simulink model "EHB_speedgoat_R2020a_V1"  (R2020a)
settings: Solver=FixedStepDiscrete  StartTime=0.0  StopTime=inf  FixedStep=0.001  RelTol=1e-3  EnableMultiTasking=on
model workspace (MAT data in the model file):
  A : Simulink.Signal (value not decoded)
  B : Simulink.Signal (value not decoded)
  C : Simulink.Signal (value not decoded)
  D : Simulink.Signal (value not decoded)
  E : Simulink.Signal (value not decoded)
  calin = [-9.96 -7.98 -5.98 -3.99 -1.994 0 1.995 3.992 5.99 7.98 9.97]
  calout = [-10 -8 -6 -4 -2 0 2 4 6 8 10]
symbols that are objects in the model workspace (value not decoded): C, D
undefined symbols (not defined in the file): Com1, none, ts_IO612
libraries: simulink x1436, xpcethercatlib x1223, yisutbxlib_utilities x256, xpcutilitieslib x156, hdlsllib x145, canmsglib x46, speedgoatlib_IO602_4 x11, speedgoatlib_IO611 x7, slrttcplib x4, CanManageLib x3, slrtlib x3, xpcseriallib x2
(part 2 of 30)

== system EHB_speedgoat_R2020a_V1/TIF_04/CB2020_3 ==
  12V_DAC_CH1 : Constant  Commented=on  Value=0  OutDataTypeStr=Inherit: Inherit via back propagation
  ADC : Subsystem  mask(simucat_adc){deviceID=0, boxNum=Box 7 (Analog Board), channel1=off, channel2=off, channel3=off, channel4=off, channel5=on, channel6=off, channel7=off, channel8=off, channel9=off, channel10=off, channel11=off, channel12=off, channel13=off, channel14=off, channel15=off, channel16=off}
      mask prompts: deviceID "Device Index:"; boxNum "Select a box:"; channel1 "1"; channel2 "2"; channel3 "3"; channel4 "4"; channel5 "5"; channel6 "6"; channel7 "7"; channel8 "8"; channel9 "9"; channel10 "10"; channel11 "11"; channel12 "12"; channel13 "13"; channel14 "14"; channel15 "15"; channel16 "16"
      mask help:
      | SimuCat系列模拟板卡驱动模块。
      | 功能：模拟量转换数字量。通道数：16
      mask TypeOptions deviceID: 0 | 1 | 2 | 3 | 4 | 5 | 6 | 7 | 8 | 9 | 10 | 11 | 12 | 13 | 14 | 15
      mask TypeOptions boxNum: Box 5 (Analog Board) | Box 6 (Analog Board) | Box 7 (Analog Board)
      mask DialogControl refreshButton Prompt: Refresh
      mask DialogControl refreshButton Callback: ystbx.mask.callbacks.refreshBoxList
      mask DialogControl selectChannel Prompt: Select channels:
      mask DialogControl Dummy Prompt: (Add text here)
      mask DialogControl channelSelectAll Prompt: Select All
      mask DialogControl channelSelectAll Callback: ystbx.mask.callbacks.selectAllChannels();
      mask DialogControl channelClearAll Prompt: Clear All
      mask DialogControl channelClearAll Callback: ystbx.mask.callbacks.clearAllChannels();
      mask DialogControl applyButton Prompt: Apply Modification
      mask DialogControl applyButton Callback: ystbx.mask.callbacks.maskApply();
      mask Display: disp('CB2020(Analog Board)\nanalog-to-digital converter\nNetwork Device 0\nBox 7 (Analog Board)');port_label('output',1,'ADC_CH5[V]');
  ADC_CH{6..16} (11 alike) : Gain  Commented=on  OutDataTypeStr=Inherit: Inherit via back propagation
  ADC_CH5 : Gain  OutDataTypeStr=Inherit: Inherit via back propagation
  AI1 : Subsystem  Commented=on
  AI2 : Subsystem  Commented=on
  AI3 : Subsystem  Commented=on
  AI4 : Subsystem  Commented=on
  DAC1 : Subsystem  mask(simucat_dac){deviceID=0, boxNum=Box 7 (Analog Board), channel1=on, channel2=off, channel3=off, channel4=off, channel5=off, channel6=off, channel7=off, channel8=off, channel9=off, channel10=off, channel11=off, channel12=off, channel13=off, channel14=off, channel15=off, channel16=off, channel17=off, channel18=off, channel19=off, channel20=off, calEnable=off, currentMode=off}
      mask prompts: deviceID "Device Index:"; boxNum "Select a box:"; channel1 "1"; channel2 "2"; channel3 "3"; channel4 "4"; channel5 "5"; channel6 "6"; channel7 "7"; channel8 "8"; channel9 "9"; channel10 "10"; channel11 "11"; channel12 "12"; channel13 "13"; channel14 "14"; channel15 "15"; channel16 "16"; channel17 "17"; channel18 "18"; channel19 "19"; channel20 "20"; calEnable "Enable DAC Calibrate"; currentMode "Apply Last 4 Channels(17~20) with Current Mode"
      mask help:
      | SimuCat系列模拟板卡驱动模块。
      | 功能：数字量转换模拟量。通道数：20
      settings: OpenFcn=open_system(gcb, 'mask');
      mask TypeOptions deviceID: 0 | 1 | 2 | 3 | 4 | 5 | 6 | 7 | 8 | 9 | 10 | 11 | 12 | 13 | 14 | 15
      mask TypeOptions boxNum: Box 5 (Analog Board) | Box 6 (Analog Board) | Box 7 (Analog Board)
      mask DialogControl refreshButton Prompt: Refresh
      mask DialogControl refreshButton Callback: ystbx.mask.callbacks.refreshBoxList
      mask DialogControl selectChannel Prompt: Select channels:
      mask DialogControl Dummy Prompt: (Add text here)
      mask DialogControl channelSelectAll Prompt: Select All
      mask DialogControl channelSelectAll Callback: ystbx.mask.callbacks.selectAllChannels();
      mask DialogControl channelClearAll Prompt: Clear All
      mask DialogControl channelClearAll Callback: ystbx.mask.callbacks.clearAllChannels();
      mask DialogControl applyButton Prompt: Apply Modification
      mask DialogControl applyButton Callback: ystbx.mask.callbacks.maskApply();
      mask Display: disp('CB2020(Analog Board)\ndigital-to-analog converter\nNetwork Device 0\nBox 7 (Analog Board)');port_label('input',1,'DAC_CH1[V]');
  Divide : Product  Inputs=*/
  Gain : Gain
  Gain{1..15} (15 alike) : Gain  Commented=on
  K : Constant  Value=6
  Sw : Subsystem
  Sw1 : Subsystem  Commented=on
  Sw10 : Subsystem  Commented=on
  Sw11 : Subsystem  Commented=on
  Sw2 : Subsystem  Commented=on
  Sw3 : Subsystem  Commented=on
  Sw4 : Subsystem  Commented=on
  Sw5 : Subsystem  Commented=on
  Sw6 : Subsystem  Commented=on
  Sw7 : Subsystem  Commented=on
  Sw8 : Subsystem  Commented=on
  Sw9 : Subsystem  Commented=on
  Terminator : Terminator
  Terminator{1..15} (15 alike) : Terminator  Commented=on
  mean1 : Subsystem
  mean10 : Subsystem  Commented=on
  mean11 : Subsystem  Commented=on
  mean12 : Subsystem  Commented=on
  mean13 : Subsystem  Commented=on
  mean14 : Subsystem  Commented=on
  mean15 : Subsystem  Commented=on
  mean16 : Subsystem  Commented=on
  mean2 : Subsystem  Commented=on
  mean3 : Subsystem  Commented=on
  mean4 : Subsystem  Commented=on
  mean5 : Subsystem  Commented=on
  mean6 : Subsystem  Commented=on
  mean7 : Subsystem  Commented=on
  mean8 : Subsystem  Commented=on
  mean9 : Subsystem  Commented=on
  tag scope: Power_5V=global
  wires:
  ADC_CH10/1 -> Gain5/1  "ADC_CH10"
  ADC_CH8/1 -> Gain3/1  "ADC_CH8"
  ADC_CH14/1 -> Gain9/1  "ADC_CH14"
  ADC_CH5/1 -> [Power_5V], Gain/1  "ADC_CH5"
  ADC_CH12/1 -> Gain7/1  "ADC_CH12"
  ADC_CH16/1 -> Gain11/1  "ADC_CH16"
  ADC_CH15/1 -> Gain10/1  "ADC_CH15"
  ADC_CH7/1 -> Gain2/1  "ADC_CH7"
  ADC_CH11/1 -> Gain6/1  "ADC_CH11"
  ADC_CH13/1 -> Gain8/1  "ADC_CH13"
  ADC_CH6/1 -> Gain1/1  "ADC_CH6"
  ADC_CH9/1 -> Gain4/1  "ADC_CH9"
  AI4/1(Cur) -> Gain15/1  "ADC_CH24"
  AI3/1(Cur) -> Gain14/1  "ADC_CH23"
  AI2/1(Cur) -> Gain13/1  "ADC_CH22"
  AI1/1(Cur) -> Gain12/1  "ADC_CH21"
  mean16/1(Vol) -> AI4/1(Vol)
  mean15/1(Vol) -> AI3/1(Vol)
  mean14/1(Vol) -> AI2/1(Vol)
  mean13/1(Vol) -> AI1/1(Vol)
  mean1/1(Vol) -> Sw/3(Vol), Sw/1(In2), Sw/2(In3)
  Sw/1(Out1) -> ADC_CH5/1
  mean2/1(Vol) -> Sw1/3(Vol), Sw1/1(In2), Sw1/2(In3)
  mean3/1(Vol) -> Sw2/3(Vol), Sw2/2(In3), Sw2/1(In2)
  mean4/1(Vol) -> Sw3/3(Vol), Sw3/2(In3), Sw3/1(In2)
  mean5/1(Vol) -> Sw4/3(Vol), Sw4/2(In3), Sw4/1(In2)
  mean6/1(Vol) -> Sw5/3(Vol), Sw5/2(In3), Sw5/1(In2)
  mean7/1(Vol) -> Sw6/3(Vol), Sw6/2(In3), Sw6/1(In2)
  mean8/1(Vol) -> Sw7/3(Vol), Sw7/2(In3), Sw7/1(In2)
  mean9/1(Vol) -> Sw9/3(Vol), Sw9/2(In3), Sw9/1(In2)
  mean10/1(Vol) -> Sw8/3(In3), Sw8/2(In2), Sw8/1(Vol)
  mean11/1(Vol) -> Sw10/3(Vol), Sw10/2(In3), Sw10/1(In2)
  mean12/1(Vol) -> Sw11/3(Vol), Sw11/2(In3), Sw11/1(In2)
  Sw11/1(Out1) -> ADC_CH16/1
  Sw10/1(Out1) -> ADC_CH15/1
  Sw8/1(Out1) -> ADC_CH14/1
  Sw9/1(Out1) -> ADC_CH13/1
  Sw7/1(Out1) -> ADC_CH12/1
  Sw6/1(Out1) -> ADC_CH11/1
  Sw5/1(Out1) -> ADC_CH10/1
  Sw4/1(Out1) -> ADC_CH9/1
  Sw3/1(Out1) -> ADC_CH8/1
  Sw2/1(Out1) -> ADC_CH7/1
  Sw1/1(Out1) -> ADC_CH6/1
  ADC/1(ADC_CH5[V]) -> mean1/1(In1)
  Gain/1 -> Terminator/1
  Gain1/1 -> Terminator1/1
  Gain2/1 -> Terminator2/1
  Gain3/1 -> Terminator3/1
  Gain4/1 -> Terminator4/1
  Gain5/1 -> Terminator5/1
  Gain11/1 -> Terminator11/1
  Gain10/1 -> Terminator10/1
  Gain9/1 -> Terminator9/1
  Gain8/1 -> Terminator8/1
  Gain7/1 -> Terminator7/1
  Gain6/1 -> Terminator6/1
  Gain15/1 -> Terminator15/1
  Gain14/1 -> Terminator14/1
  Gain13/1 -> Terminator13/1
  Gain12/1 -> Terminator12/1
  K/1 -> Divide/2
  [PowerOn_Off] -> Divide/1  "12V_DAC_CH1"
  Divide/1 -> DAC1/1(DAC_CH1[V])  "12V_DAC_CH1"

== system EHB_speedgoat_R2020a_V1/YS5002/YS5002_M_PowerCtrl ==
  note: 1、模拟量控制比例要看具体电源输出范围计算，
      |      例如：电源0~80V对应DAC的0~10V，设定12V时实际下发给DAC的是1/8*1000mV。
      | 2、Rly通过哪两个继电器去控制KL30,15要确认下机柜具体的实际接线，一般是Rly1,2。
      | 3、OnOff一般接SwitchA，通过下降沿去触发。
  YS5002_M : Inport
  Enable : EnablePort
  Bus Selector : BusSelector  OutputSignals=PS1,PS2,PS3,PS4
  CAN Pack : canmsglib/CAN Pack  MsgList=(none)  MsgName=PowerSet  MsgIDType=Standard (11-bit identifier)  MsgIdentifier=1852  MsgLength=8  Remote=off  ApplyMinMax=off  BusOutput=on  SignalInfo={ 'ADC1_Calibration_en', '52', '1', 'BE', 'unsigned', 'Standard', '0', '1', '0', '0', '1'; 'ADC2_Calibration_en', '53', '1', 'BE', 'unsigned', 'Standard', '0', '1', '0', '0', '1'; 'ADCorDAC_Calibration_Data', '56', '12', 'BE', 'unsigned', 'Standard', '0', '1', '0', '500', '1500'; 'Calibration_en', '14', '1', 'BE', 'unsigned', 'Standard', '0', '1', '0', '0', '1'; 'DAC1_Set', '24', '16', 'BE', 'unsigned', 'Standard', '0', '1', '0', '0', '10000'; 'DAC2_Set', '40', '16', 'BE', 'unsigned', 'Standard', '0', '1', '0', '0', '10000'; 'DCA1_Calibration_en', '54', '1', 'BE', 'unsigned', 'Standard', '0', '1', '0', '0', '1'; 'DCA2_Calibration_en', '55', '1', 'BE', 'unsigned', 'Standard', '0', '1', '0', '0', '1'; 'Rly1_Ctrl', '11', '1', 'BE', 'unsigned', 'Standard', '0', '1', '0', '0', '1'; 'Rly2_Ctrl', '10', '1', 'BE', 'unsigned', 'Standard', '0', '1', '0', '0', '1'; 'Rly3_Ctrl', '9', '1', 'BE', 'unsigned', 'Standard', '0', '1', '0', '0', '1'; 'Rly4_Ctrl', '8', '1', 'BE', 'unsigned', 'Standard', '0', '1', '0', '0', '1'; 'Slot', '0', '8', 'BE', 'unsigned', 'Standard', '0', '1', '0', '0', '15'; 'SwitchA', '12', '1', 'BE', 'unsigned', 'Standard', '0', '1', '0', '0', '1'; 'SwitchB', '13', '1', 'BE', 'unsigned', 'Standard', '0', '1', '0', '0', '1'; 'Trig_en', '15', '1', 'BE', 'unsigned', 'Standard', '0', '1', '0', '0', '1' }
      settings: SourceProductBaseCode=ME,XP,VN  DataFormat=manually specified signals
  CANDataPack_ToUDP : Subsystem
  Cur : Constant  Value=0  OutDataTypeStr=Inherit: Inherit via back propagation
  Gain1 : Gain  Gain=1000/8
  Gain2 : Gain  Gain=1000/8
  InternalUse : Constant  Value=0  OutDataTypeStr=Inherit: Inherit via back propagation
  InternalUse1 : Constant  Value=0  OutDataTypeStr=Inherit: Inherit via back propagation
  Logical Operator : Logic  Operator=NOT  AllPortsSameDT=off  OutDataTypeStr=boolean
  Solt : Constant  Value=0
  Sw : Constant  Value=0  OutDataTypeStr=Inherit: Inherit via back propagation
  SwitchB : Constant  Value=0  OutDataTypeStr=Inherit: Inherit via back propagation
  Trig_en : Constant  Value=0  OutDataTypeStr=Inherit: Inherit via back propagation
  Vol : Constant  Value=0  OutDataTypeStr=Inherit: Inherit via back propagation
  Output : Outport
  wires:
  Vol/1 -> Gain2/1  "VoltSet"
  Cur/1 -> Gain1/1  "CurrLimSet"
  InternalUse/1 -> CAN Pack/4, CAN Pack/3, CAN Pack/2, CAN Pack/1
  YS5002_M/1 -> Bus Selector/1
  Bus Selector/1 -> [PS1]  "<PS1>"
  Bus Selector/2 -> [PS2]  "<PS2>"
  Bus Selector/3 -> [PS3]  "<PS3>"
  Solt/1 -> CAN Pack/13
  [PS1] -> CAN Pack/9
  [PS2] -> CAN Pack/10
  Trig_en/1 -> CAN Pack/16  "Trig_en"
  Gain2/1 -> CAN Pack/5  "DAC1_Set"
  Gain1/1 -> CAN Pack/6  "DAC2_Set"
  InternalUse1/1 -> CAN Pack/8, CAN Pack/7
  Bus Selector/4 -> [PS4]  "<PS4>"
  SwitchB/1 -> CAN Pack/14
  Logical Operator/1 -> CAN Pack/15
  Sw/1 -> Logical Operator/1  "Sw"
  [PS3] -> CAN Pack/11
  [PS4] -> CAN Pack/12
  CAN Pack/1 -> CANDataPack_ToUDP/1(In1)
  CANDataPack_ToUDP/1(Out1) -> Output/1

== system EHB_speedgoat_R2020a_V1/保留/IO602 ==
  CAN Pack : canmsglib/CAN Pack  MsgList=(none)  MsgName=CAN Msg  MsgIDType=Standard (11-bit identifier)  MsgIdentifier=100  MsgLength=8  Remote=off  ApplyMinMax=off  BusOutput=off  SignalInfo={'Signal1','0','64','LE','double','Standard','0','1','0','-Inf','Inf'}
      settings: SourceProductBaseCode=ME,VN  DataFormat=manually specified signals
  CAN Pack1 : canmsglib/CAN Pack  MsgList=(none)  MsgName=CAN Msg  MsgIDType=Standard (11-bit identifier)  MsgIdentifier=101  MsgLength=8  Remote=off  ApplyMinMax=off  BusOutput=off  SignalInfo={'Signal1','0','64','LE','double','Standard','0','1','0','-Inf','Inf'}
      settings: SourceProductBaseCode=ME,VN  DataFormat=manually specified signals
  CAN Pack2 : canmsglib/CAN Pack  MsgList=(none)  MsgName=CAN Msg  MsgIDType=Standard (11-bit identifier)  MsgIdentifier=102  MsgLength=8  Remote=off  ApplyMinMax=off  BusOutput=off  SignalInfo={'Signal1','0','64','LE','double','Standard','0','1','0','-Inf','Inf'}
      settings: SourceProductBaseCode=ME,VN  DataFormat=manually specified signals
  CAN Pack3 : canmsglib/CAN Pack  MsgList=(none)  MsgName=CAN Msg  MsgIDType=Standard (11-bit identifier)  MsgIdentifier=100  MsgLength=8  Remote=off  ApplyMinMax=off  BusOutput=off  SignalInfo={'Signal1','0','64','LE','double','Standard','0','1','0','-Inf','Inf'}
      settings: SourceProductBaseCode=ME,VN  DataFormat=manually specified signals
  CAN Pack4 : canmsglib/CAN Pack  MsgList=(none)  MsgName=CAN Msg  MsgIDType=Standard (11-bit identifier)  MsgIdentifier=101  MsgLength=8  Remote=off  ApplyMinMax=off  BusOutput=off  SignalInfo={'Signal1','0','64','LE','double','Standard','0','1','0','-Inf','Inf'}
      settings: SourceProductBaseCode=ME,VN  DataFormat=manually specified signals
  CAN Pack5 : canmsglib/CAN Pack  MsgList=(none)  MsgName=CAN Msg  MsgIDType=Standard (11-bit identifier)  MsgIdentifier=102  MsgLength=8  Remote=off  ApplyMinMax=off  BusOutput=off  SignalInfo={'Signal1','0','64','LE','double','Standard','0','1','0','-Inf','Inf'}
      settings: SourceProductBaseCode=ME,VN  DataFormat=manually specified signals
  CAN Read Loop - Port 1 : Subsystem  TreatAsAtomicUnit=on
  CAN Read Loop - Port 3 : Subsystem  TreatAsAtomicUnit=on
  CAN Write : speedgoatlib_IO602_4/Legacy/CAN Write  id=1  ts=-1  channel=1  messageType=CAN  BusInput=off  enableStatusPort=off  canType=CAN (HS)  initValues=[602 1 -1 0 1 1 0 0]
      settings: SourceProductName=Simulink Real-Time: Speedgoat I/O Blockset
  CAN Write1 : speedgoatlib_IO602_4/Legacy/CAN Write  id=1  ts=-1  channel=1  messageType=CAN  BusInput=off  enableStatusPort=off  canType=CAN (HS)  initValues=[602 1 -1 0 1 1 0 0]
      settings: SourceProductName=Simulink Real-Time: Speedgoat I/O Blockset
  CAN Write2 : speedgoatlib_IO602_4/Legacy/CAN Write  id=1  ts=-1  channel=1  messageType=CAN  BusInput=off  enableStatusPort=off  canType=CAN (HS)  initValues=[602 1 -1 0 1 1 0 0]
      settings: SourceProductName=Simulink Real-Time: Speedgoat I/O Blockset
  CAN Write3 : speedgoatlib_IO602_4/Legacy/CAN Write  id=1  ts=-1  channel=3  messageType=CAN  BusInput=off  enableStatusPort=off  canType=CAN (HS)  initValues=[602 1 -1 2 1 1 0 0]
      settings: SourceProductName=Simulink Real-Time: Speedgoat I/O Blockset
  CAN Write4 : speedgoatlib_IO602_4/Legacy/CAN Write  id=1  ts=-1  channel=3  messageType=CAN  BusInput=off  enableStatusPort=off  canType=CAN (HS)  initValues=[602 1 -1 2 1 1 0 0]
      settings: SourceProductName=Simulink Real-Time: Speedgoat I/O Blockset
  CAN Write5 : speedgoatlib_IO602_4/Legacy/CAN Write  id=1  ts=-1  channel=3  messageType=CAN  BusInput=off  enableStatusPort=off  canType=CAN (HS)  initValues=[602 1 -1 2 1 1 0 0]
      settings: SourceProductName=Simulink Real-Time: Speedgoat I/O Blockset
  Mux : Mux  Inputs=3
  Mux2 : Mux  Inputs=3
  RX Sample Time : Constant  SampleTime=ts_IO612
  RX Sample Time1 : Constant  SampleTime=ts_IO612
  "Scope " : slrtlib/Displays and Logging/Scope   scopeno=1  scopetype=Target  autostart=on  viewmode=Graphical redraw  formatstr='%15.6f'  grid=on  ylimits=[0,0]  nosamples=250  noprepostsamples=0  interleave=1  triggermode=FreeRun  triggersignal=1  trigsignalfromport=off  triggerlevel=0.0  triggerslope=Rising  triggerscope=1  triggersample=0  filename=data.dat  mode=Lazy  writesize=512  autorestart=off  dynamicfilemode=off  maxwritefilesize=512*1024^2
  Scope 1 : slrtlib/Displays and Logging/Scope   scopeno=2  scopetype=Target  autostart=on  viewmode=Graphical redraw  formatstr='%15.6f'  grid=on  ylimits=[0,0]  nosamples=250  noprepostsamples=0  interleave=1  triggermode=FreeRun  triggersignal=1  trigsignalfromport=off  triggerlevel=0.0  triggerslope=Rising  triggerscope=1  triggersample=0  filename=data.dat  mode=Lazy  writesize=512  autorestart=off  dynamicfilemode=off  maxwritefilesize=512*1024^2
  Sine Wave : Sin  Amplitude=10  Frequency=2*pi*10  SampleTime=ts_IO612
  Sine Wave1 : Sin  Amplitude=20  Frequency=2*pi*10  SampleTime=ts_IO612
  Sine Wave2 : Sin  Amplitude=30  Frequency=2*pi*10  SampleTime=ts_IO612
  Sine Wave3 : Sin  Amplitude=10  Frequency=2*pi*10  SampleTime=ts_IO612
  Sine Wave4 : Sin  Amplitude=20  Frequency=2*pi*10  SampleTime=ts_IO612
  Sine Wave5 : Sin  Amplitude=30  Frequency=2*pi*10  SampleTime=ts_IO612
  wires:
  Mux/1 -> "Scope "/1  "IO602Can1-2"
  CAN Read Loop - Port 3/1(ID100_Signal1) -> Mux/1
  CAN Read Loop - Port 3/3(ID102_Signal1) -> Mux/3
  CAN Read Loop - Port 3/2(ID101_Signal1) -> Mux/2
  RX Sample Time/1 -> CAN Read Loop - Port 3/1(SampleTime)
  Sine Wave1/1 -> CAN Pack1/1
  Sine Wave/1 -> CAN Pack/1
  Sine Wave2/1 -> CAN Pack2/1
  CAN Pack/1 -> CAN Write/1
  CAN Pack1/1 -> CAN Write1/1
  CAN Pack2/1 -> CAN Write2/1
  CAN Pack5/1 -> CAN Write5/1
  CAN Pack4/1 -> CAN Write4/1
  CAN Pack3/1 -> CAN Write3/1
  Sine Wave5/1 -> CAN Pack5/1
  Sine Wave3/1 -> CAN Pack3/1
  Sine Wave4/1 -> CAN Pack4/1
  RX Sample Time1/1 -> CAN Read Loop - Port 1/1(SampleTime)
  CAN Read Loop - Port 1/2(ID101_Signal1) -> Mux2/2
  CAN Read Loop - Port 1/3(ID102_Signal1) -> Mux2/3
  CAN Read Loop - Port 1/1(ID100_Signal1) -> Mux2/1
  Mux2/1 -> Scope 1/1  "IO602Can3-4"

== system EHB_speedgoat_R2020a_V1/保留/IO611 ==
  note: PORT 1 - TX
  note: PORT 1 - TX
  note: PORT 2 - RX
  note: PORT 2 - RX
  "Byte Packing " : xpcutilitieslib/Byte Packing   MaskPackedDataType=uint8  MaskUnpackedDataTypes={'uint8','uint8'}  MaskAlignment=1
  CAN Pack : canmsglib/CAN Pack  MsgList=(none)  MsgName=CAN Msg  MsgIDType=Standard (11-bit identifier)  MsgIdentifier=100  MsgLength=8  Remote=off  ApplyMinMax=off  BusOutput=off  SignalInfo={'Signal1','0','64','LE','double','Standard','0','1','0','-Inf','Inf'}
      settings: SourceProductBaseCode=ME,VN  DataFormat=manually specified signals
  CAN Pack1 : canmsglib/CAN Pack  MsgList=(none)  MsgName=CAN Msg  MsgIDType=Standard (11-bit identifier)  MsgIdentifier=101  MsgLength=8  Remote=off  ApplyMinMax=off  BusOutput=off  SignalInfo={'Signal1','0','64','LE','double','Standard','0','1','0','-Inf','Inf'}
      settings: SourceProductBaseCode=ME,VN  DataFormat=manually specified signals
  CAN Pack2 : canmsglib/CAN Pack  MsgList=(none)  MsgName=CAN Msg  MsgIDType=Standard (11-bit identifier)  MsgIdentifier=102  MsgLength=8  Remote=off  ApplyMinMax=off  BusOutput=off  SignalInfo={'Signal1','0','64','LE','double','Standard','0','1','0','-Inf','Inf'}
      settings: SourceProductBaseCode=ME,VN  DataFormat=manually specified signals
  CAN Read Loop - Port 3 : Subsystem  TreatAsAtomicUnit=on
  CAN Write : speedgoatlib_IO611/Legacy/CAN/CAN Write  id=1  sampleTime=-1  portSelection=1  messageType=CAN  BusInput=off  enaStatusPort=off  protl=IO611  ptIdx=0  isFDMod=1
      settings: SourceProductName=Simulink Real-Time: Speedgoat I/O Blockset
  CAN Write1 : speedgoatlib_IO611/Legacy/CAN/CAN Write  id=1  sampleTime=-1  portSelection=1  messageType=CAN  BusInput=off  enaStatusPort=off  protl=IO611  ptIdx=0  isFDMod=1
      settings: SourceProductName=Simulink Real-Time: Speedgoat I/O Blockset
  CAN Write2 : speedgoatlib_IO611/Legacy/CAN/CAN Write  id=1  sampleTime=-1  portSelection=1  messageType=CAN  BusInput=off  enaStatusPort=off  protl=IO611  ptIdx=0  isFDMod=1
      settings: SourceProductName=Simulink Real-Time: Speedgoat I/O Blockset
  Constant1 : Constant  Value=80  OutDataTypeStr=uint8
  Data Type Conversion : DataTypeConversion
  Gain : Gain
  "LIN Master Write v2 " : speedgoatlib_IO611/Legacy/LIN/LIN Master Write v2   id=1  sampleTime=-1  portSelection=3  messageType=RAW  linVersion=LIN 2.X  protIdent=0  dlc=2  dummy1=dummy for default msg data used for slave write block  protl=IO611  ptIdx=2  isSlv=0  isEnhcdChksum=1  qtyMsgBlkLIN=1
      settings: SourceProductName=Simulink Real-Time: Speedgoat I/O Blockset
  "LIN Slave Read v2 " : speedgoatlib_IO611/Legacy/LIN/LIN Slave Read v2   id=1  sampleTime=-1  portSelection=4  enaUpdateState=off  enaMsgType=off  enaDataOverrun=off  enaTimeStampe=off  messageType=RAW  linVersion=LIN 2.X  protIdent=0  dlc=2  protl=IO611  ptIdx=3  isSlv=1  isEnhcdChksum=1  qtyMsgBlkLIN=1
      settings: SourceProductName=Simulink Real-Time: Speedgoat I/O Blockset
  Mux : Mux  Inputs=3
  Pulse Generator : DiscretePulseGenerator  PulseType=Time based  Amplitude=20  Period=10  PulseWidth=50
  RX Sample Time : Constant  SampleTime=ts_IO612
  "Scope " : slrtlib/Displays and Logging/Scope   scopeno=3  scopetype=Target  autostart=on  viewmode=Graphical redraw  formatstr='%15.6f'  grid=on  ylimits=[0,0]  nosamples=250  noprepostsamples=0  interleave=1  triggermode=FreeRun  triggersignal=1  trigsignalfromport=off  triggerlevel=0.0  triggerslope=Rising  triggerscope=1  triggersample=0  filename=data.dat  mode=Lazy  writesize=512  autorestart=off  dynamicfilemode=off  maxwritefilesize=512*1024^2
  Sine Wave : Sin  Amplitude=10  Frequency=2*pi*10  SampleTime=ts_IO612
  Sine Wave1 : Sin  Amplitude=20  Frequency=2*pi*10  SampleTime=ts_IO612
  Sine Wave2 : Sin  Amplitude=30  Frequency=2*pi*10  SampleTime=ts_IO612
  Terminator : Terminator
  wires:
  Constant1/1 -> "Byte Packing "/1  "LIN_Data1"
  Pulse Generator/1 -> Data Type Conversion/1
  "Byte Packing "/1 -> "LIN Master Write v2 "/1
  "LIN Slave Read v2 "/1 -> Gain/1  "IO611_LIN_Rx"
  CAN Pack1/1 -> CAN Write1/1
  Sine Wave2/1 -> CAN Pack2/1
  Sine Wave/1 -> CAN Pack/1
  CAN Read Loop - Port 3/3(ID102_Signal1) -> Mux/3
  Sine Wave1/1 -> CAN Pack1/1
  RX Sample Time/1 -> CAN Read Loop - Port 3/1(SampleTime)
  CAN Pack2/1 -> CAN Write2/1
  CAN Read Loop - Port 3/2(ID101_Signal1) -> Mux/2
  CAN Pack/1 -> CAN Write/1
  CAN Read Loop - Port 3/1(ID100_Signal1) -> Mux/1
  Mux/1 -> "Scope "/1  "IO611"
  Data Type Conversion/1 -> "Byte Packing "/2  "LIN_Data2"
  Gain/1 -> Terminator/1

== system EHB_speedgoat_R2020a_V1/保留/RS232 ==
  Baseboard Serial F2 : xpcseriallib/Mainboard/Baseboard Serial F  group=FIFO Setup  port=1  irqnum=4  saddr1=0x3f8  saddr2=0x3e8  config=Com1/none  baud1=115200  parity1=None  ndata1=8  nstop1=1  fifomode1=16 deep  rlevel1=half full  automode1=on  xmtfifosize1=1024  xmtdatatype1=count+16 bit uint  rcvfifosize1=1024  baud2=115200  parity2=None  ndata2=8  nstop2=1  fifomode2=16 deep  rlevel2=half full  automode2=off  xmtfifosize2=1024  xmtdatatype2=8 bit uint null terminated  rcvfifosize2=1024
      settings: SourceProductBaseCode=XP
  "Byte Packing " : xpcutilitieslib/Byte Packing   MaskPackedDataType=uint8  MaskUnpackedDataTypes={'double'}  MaskAlignment=1
  Constant1 : Constant  Value=10
  Data Type Conversion : DataTypeConversion  OutDataTypeStr=uint16
  Data Type Conversion1 : DataTypeConversion  OutDataTypeStr=double
  "FIFO read " : xpcseriallib/FIFO read   maxsize=16  minsize=8  usedelimiter=off  delimiter=13  outputtype=count+16 bit uint  enable=off  enableout=off  sampletime=-1
      settings: SourceProductBaseCode=XP
  Gain : Gain
  Gain1 : Gain
  Ground3 : Ground
  Mux : Mux  Inputs=2
  Selector : Selector  InputPortWidth=17  IndexOptions=Index vector (dialog)  Indices=[2:9]  OutputSizes=1
  Terminator : Terminator
  Terminator1 : Terminator
  Terminator4 : Terminator
  Width : Width  DataType=uint16
  wires:
  "FIFO read "/1 -> Gain1/1, Selector/1  "FIOFO_Received_Data"
  Baseboard Serial F2/2 -> Terminator4/1
  Constant1/1 -> "Byte Packing "/1
  Ground3/1 -> Baseboard Serial F2/2
  Mux/1 -> Baseboard Serial F2/1  "RS232_Send"
  Width/1 -> Mux/1
  Data Type Conversion/1 -> Mux/2
  "Byte Packing "/1 -> Width/1, Data Type Conversion/1  "pack"
  Baseboard Serial F2/1 -> "FIFO read "/1
  Selector/1 -> Data Type Conversion1/1
  Data Type Conversion1/1 -> Gain/1  "RS232ReceiveData"
  Gain/1 -> Terminator/1
  Gain1/1 -> Terminator1/1

== system EHB_speedgoat_R2020a_V1/保留/TIF_01 ==
  YS4020_M_2 : Subsystem

== system EHB_speedgoat_R2020a_V1/保留/TIF_02 ==
  CB3012_01 : Subsystem

== system EHB_speedgoat_R2020a_V1/保留/TIF_03 ==
  CB1032_3 : Subsystem
  CB1032_4 : Subsystem

== system EHB_speedgoat_R2020a_V1/保留/TIF_06 ==
  CB1032_1 : Subsystem
  CB1032_2 : Subsystem
  YS4020_M_1 : Subsystem

== system EHB_speedgoat_R2020a_V1/保留/YS4008 ==
  YS4008_M_1 : Subsystem
  YS4008_M_2 : Subsystem
  YS4008_M_3 : Subsystem
  YS4008_M_4 : Subsystem
  YS4008_M_5 : Subsystem
  YS4008_M_6 : Subsystem

== system EHB_speedgoat_R2020a_V1/保留/YS7501_M ==
  Bitwise OR : simulink/Logic and Bit Operations/Bitwise Operator  logicop=OR  UseBitMask=off  BitMask=bin2dec('11011001')  BitMaskRealWorld=Stored Integer
  Constant{,1..15} (16 alike) : Constant  Value=0
  Detect Change : simulink/Logic and Bit Operations/Detect Change  vinit=0  OutDataTypeStr=boolean
  HVRealy_Set : Subsystem
  Mux : Mux  Inputs=16
  tag scope: YS7501_M=global
  wires:
  Constant1/1 -> HVRealy_Set/2(RLY2), Mux/2
  Constant3/1 -> HVRealy_Set/4(RLY4), Mux/4
  Constant2/1 -> HVRealy_Set/3(RLY3), Mux/3
  Constant/1 -> HVRealy_Set/1(RLY1), Mux/1
  Mux/1 -> Detect Change/1
  Constant4/1 -> HVRealy_Set/5(RLY5), Mux/5
  Constant5/1 -> HVRealy_Set/6(RLY6), Mux/6
  Constant7/1 -> HVRealy_Set/8(RLY8), Mux/8
  Constant8/1 -> HVRealy_Set/9(RLY9), Mux/9
  Constant9/1 -> HVRealy_Set/10(RLY10), Mux/10
  Constant10/1 -> HVRealy_Set/11(RLY11), Mux/11
  Constant11/1 -> HVRealy_Set/12(RLY12), Mux/12
  Constant12/1 -> HVRealy_Set/13(RLY13), Mux/13
  Constant13/1 -> Mux/14, HVRealy_Set/14(RLY14)
  Constant14/1 -> Mux/15, HVRealy_Set/15(RLY15)
  Constant15/1 -> Mux/16, HVRealy_Set/16(RLY16)
  Constant6/1 -> HVRealy_Set/7(RLY7), Mux/7
  Detect Change/1 -> Bitwise OR/1  "HVRealy_Ctrl_Trigger"
  Bitwise OR/1 -> HVRealy_Set/Trigger
  HVRealy_Set/1(Output) -> [YS7501_M]

== system EHB_speedgoat_R2020a_V1/CAN_Rec/CAN Receive/CAN_Msg_0x125 ==
  CAN Msg : Inport
  Enable : EnablePort
  Bus Creator : BusCreator  Inputs=6
  Can Unpack : canmsglib/CAN Unpack  CANdbFile=D:\Matlab\EHB_Prj\data\DBC\wushuadianji_20230612.dbc  MsgList=EHB_BrakingResponse  MsgName=EHB_BrakingResponse  MsgIDType=Standard (11-bit identifier)  MsgIdentifier=293  MsgLength=8  SignalInfo={'ActualPressure','8','8','BE','unsigned','Standard','0','0.1','0','-Inf','Inf';'BrakeCondition','1','2','BE','unsigned','Standard','0','1','0','-Inf','Inf';'Checksum','56','8','BE','unsigned','Standard','0','1','0','-Inf','Inf';'EHBFaultLevel','3','4','BE','unsigned','Standard','0','1','0','-Inf','Inf';'EHBStatus','0','1','BE','unsigned','Standard','0','1','0','-Inf','Inf';'RollingCounter','52','4','BE','unsigned','Standard','0','1','0','-Inf','Inf'}  IDPort=off  TimestampPort=off  ErrorPort=off  RemotePort=off  LengthPort=off  StatusPort=off  ApplyMinMax=off
      settings: SourceProductBaseCode=ME,VN  DataFormat=CANdb specified signals
  EHB_0125h_AliveCounter : DataTypeConversion
  EHB_0125h_CheckSUM : DataTypeConversion
  EHB_ActualPressure : DataTypeConversion
  EHB_BrakeCondition : DataTypeConversion
  EHB_EHBFaultLevel : DataTypeConversion
  EHB_Status : DataTypeConversion
  CAN_Msg_0x125 : Outport
  wires:
  Bus Creator/1 -> CAN_Msg_0x125/1  "CAN_Msg_0x125"
  EHB_0125h_CheckSUM/1 -> Bus Creator/3  "EHB_0125h_CheckSUM"
  Can Unpack/3 -> EHB_0125h_CheckSUM/1
  EHB_BrakeCondition/1 -> Bus Creator/2  "EHB_BrakeCondition"
  Can Unpack/2 -> EHB_BrakeCondition/1
  EHB_ActualPressure/1 -> Bus Creator/1  "EHB_ActualPressure"
  Can Unpack/1 -> EHB_ActualPressure/1
  CAN Msg/1 -> Can Unpack/1
  Can Unpack/4 -> EHB_EHBFaultLevel/1
  Can Unpack/5 -> EHB_Status/1
  Can Unpack/6 -> EHB_0125h_AliveCounter/1
  EHB_EHBFaultLevel/1 -> Bus Creator/4  "EHB_EHBFaultLevel"
  EHB_Status/1 -> Bus Creator/5  "EHB_Status"
  EHB_0125h_AliveCounter/1 -> Bus Creator/6  "EHB_0125h_AliveCounter"

== system EHB_speedgoat_R2020a_V1/CAN_Rec/CAN Receive/CAN_Msg_0x126 ==
  CAN Msg : Inport
  Enable : EnablePort
  Bus Creator : BusCreator  Inputs=22
  Can Unpack : canmsglib/CAN Unpack  CANdbFile=D:\Matlab\EHB_Prj\data\DBC\wushuadianji_20230612.dbc  MsgList=EHB_Diagnostics  MsgName=EHB_Diagnostics  MsgIDType=Standard (11-bit identifier)  MsgIdentifier=294  MsgLength=8  SignalInfo={'BrkReqWarn','0','1','BE','unsigned','Standard','0','1','0','-Inf','Inf';'CANBusOff','12','1','BE','unsigned','Standard','0','1','0','-Inf','Inf';'EHB_HardwareVersion','56','8','BE','unsigned','Standard','0','1','0','-Inf','Inf';'EHB_SoftwareVersion','48','8','BE','unsigned','Standard','0','1','0','-Inf','Inf';'ISnsrFlt','14','1','BE','unsigned','Standard','0','1','0','-Inf','Inf';'LoadMismatchFlt','11','1','BE','unsigned','Standard','0','1','0','-Inf','Inf';'MotPosnFlt','19','1','BE','unsigned','Standard','0','1','0','-Inf','Inf';'NTCFltLv1','3','1','BE','unsigned','Standard','0','1','0','-Inf','Inf';'NTCFltLv2','4','1','BE','unsigned','Standard','0','1','0','-Inf','Inf';'OverIFlt','13','1','BE','unsigned','Standard','0','1','0','-Inf','Inf';'OverTempWarn','6','1','BE','unsigned','Standard','0','1','0','-Inf','Inf';'PCtrlVibLv1','2','1','BE','unsigned','Standard','0','1','0','-Inf','Inf';'PCtrlVibLv2','10','1','BE','unsigned','Standard','0','1','0','-Inf','Inf';'PFolwFltLv1','1','1','BE','unsigned','Standard','0','1','0','-Inf','Inf';'PFolwFltLv2','9','1','BE','unsigned','Standard','0','1','0','-Inf','Inf';'PSnsrFlt','5','1','BE','unsigned','Standard','0','1','0','-Inf','Inf';'PwrDrvrFlt','18','1','BE','unsigned','Standard','0','1','0','-Inf','Inf';'PwrSwtFlt','17','1','BE','unsigned','Standard','0','1','0','-Inf','Inf';'USplyHighLv1','8','1','BE','unsigned','Standard','0','1','0','-Inf','Inf';'USplyHighLv2','16','1','BE','unsigned','Standard','0','1','0','-Inf','Inf';'USplyLowLv1','7','1','BE','unsigned','Standard','0','1','0','-Inf','Inf';'USplyLowLv2','15','1','BE','unsigned','Standard','0','1','0','-Inf','Inf'}  IDPort=off  TimestampPort=off  ErrorPort=off  RemotePort=off  LengthPort=off  StatusPort=off  ApplyMinMax=off
      settings: SourceProductBaseCode=ME,VN  DataFormat=CANdb specified signals
  EHB_BrkReqWarn : DataTypeConversion
  EHB_CANBusOff : DataTypeConversion
  EHB_HardwareVersion : DataTypeConversion
  EHB_ISnsrFlt : DataTypeConversion
  EHB_LoadMismatchFlt : DataTypeConversion
  EHB_MotPosnFlt : DataTypeConversion
  EHB_NTCFltLv1 : DataTypeConversion
  EHB_NTCFltLv2 : DataTypeConversion
  EHB_OverIFlt : DataTypeConversion
  EHB_OverTempWarn : DataTypeConversion
  EHB_PCtrlVibLv1 : DataTypeConversion
  EHB_PCtrlVibLv2 : DataTypeConversion
  EHB_PFolwFltLv1 : DataTypeConversion
  EHB_PFolwFltLv2 : DataTypeConversion
  EHB_PSnsrFlt : DataTypeConversion
  EHB_PwrDrvrFlt : DataTypeConversion
  EHB_PwrSwtFlt : DataTypeConversion
  EHB_SoftwareVersion : DataTypeConversion
  EHB_USplyHighLv1 : DataTypeConversion
  EHB_USplyHighLv2 : DataTypeConversion
  EHB_USplyLowLv1 : DataTypeConversion
  EHB_USplyLowLv2 : DataTypeConversion
  CAN_Msg_0x126 : Outport
  wires:
  EHB_LoadMismatchFlt/1 -> Bus Creator/6  "EHB_LoadMismatchFlt"
  EHB_ISnsrFlt/1 -> Bus Creator/5  "EHB_ISnsrFlt"
  EHB_SoftwareVersion/1 -> Bus Creator/4  "EHB_SoftwareVersion"
  Can Unpack/6 -> EHB_LoadMismatchFlt/1
  Can Unpack/5 -> EHB_ISnsrFlt/1
  Can Unpack/4 -> EHB_SoftwareVersion/1
  CAN Msg/1 -> Can Unpack/1
  Can Unpack/1 -> EHB_BrkReqWarn/1
  EHB_BrkReqWarn/1 -> Bus Creator/1  "EHB_BrkReqWarn"
  Can Unpack/2 -> EHB_CANBusOff/1
  EHB_CANBusOff/1 -> Bus Creator/2  "EHB_CANBusOff"
  Can Unpack/3 -> EHB_HardwareVersion/1
  EHB_HardwareVersion/1 -> Bus Creator/3  "EHB_HardwareVersion"
  Bus Creator/1 -> CAN_Msg_0x126/1  "CAN_Msg_0x126"
  Can Unpack/7 -> EHB_MotPosnFlt/1
  Can Unpack/8 -> EHB_NTCFltLv1/1
  Can Unpack/9 -> EHB_NTCFltLv2/1
  Can Unpack/10 -> EHB_OverIFlt/1
  Can Unpack/11 -> EHB_OverTempWarn/1
  Can Unpack/12 -> EHB_PCtrlVibLv1/1
  Can Unpack/13 -> EHB_PCtrlVibLv2/1
  Can Unpack/14 -> EHB_PFolwFltLv1/1
  Can Unpack/15 -> EHB_PFolwFltLv2/1
  Can Unpack/16 -> EHB_PSnsrFlt/1
  Can Unpack/17 -> EHB_PwrDrvrFlt/1
  Can Unpack/18 -> EHB_PwrSwtFlt/1
  Can Unpack/19 -> EHB_USplyHighLv1/1
  Can Unpack/20 -> EHB_USplyHighLv2/1
  Can Unpack/21 -> EHB_USplyLowLv1/1
  Can Unpack/22 -> EHB_USplyLowLv2/1
  EHB_MotPosnFlt/1 -> Bus Creator/7  "EHB_MotPosnFlt"
  EHB_NTCFltLv1/1 -> Bus Creator/8  "EHB_NTCFltLv1"
  EHB_NTCFltLv2/1 -> Bus Creator/9  "EHB_NTCFltLv2"
  EHB_OverIFlt/1 -> Bus Creator/10  "EHB_OverIFlt"
  EHB_OverTempWarn/1 -> Bus Creator/11  "EHB_OverTempWarn"
  EHB_PCtrlVibLv1/1 -> Bus Creator/12  "EHB_PCtrlVibLv1"
  EHB_PCtrlVibLv2/1 -> Bus Creator/13  "EHB_PCtrlVibLv2"
  EHB_PFolwFltLv1/1 -> Bus Creator/14  "EHB_PFolwFltLv1"
  EHB_PFolwFltLv2/1 -> Bus Creator/15  "EHB_PFolwFltLv2"
  EHB_PSnsrFlt/1 -> Bus Creator/16  "EHB_PSnsrFlt"
  EHB_PwrDrvrFlt/1 -> Bus Creator/17  "EHB_PwrDrvrFlt"
  EHB_PwrSwtFlt/1 -> Bus Creator/18  "EHB_PwrSwtFlt"
  EHB_USplyHighLv1/1 -> Bus Creator/19  "EHB_USplyHighLv1"
  EHB_USplyHighLv2/1 -> Bus Creator/20  "EHB_USplyHighLv2"
  EHB_USplyLowLv1/1 -> Bus Creator/21  "EHB_USplyLowLv1"
  EHB_USplyLowLv2/1 -> Bus Creator/22  "EHB_USplyLowLv2"

== system EHB_speedgoat_R2020a_V1/CAN_Rec/CAN Receive/CAN_Msg_0x127 ==
  CAN Msg : Inport
  Enable : EnablePort
  Bus Creator : BusCreator  Inputs=8
  Can Unpack : canmsglib/CAN Unpack  CANdbFile=D:\Matlab\EHB_Prj\data\DBC\wushuadianji_20230612.dbc  MsgList=EHB_WhlSpd_Info  MsgName=EHB_WhlSpd_Info  MsgIDType=Standard (11-bit identifier)  MsgIdentifier=295  MsgLength=8  SignalInfo={'WhlFLSpd','10','14','BE','unsigned','Standard','0','1','0','-Inf','Inf';'WhlFLSpdVld','8','2','BE','unsigned','Standard','0','1','0','-Inf','Inf';'WhlFRSpd','26','14','BE','unsigned','Standard','0','1','0','-Inf','Inf';'WhlFRSpdVld','24','2','BE','unsigned','Standard','0','1','0','-Inf','Inf';'WhlRLSpd','42','14','BE','unsigned','Standard','0','1','0','-Inf','Inf';'WhlRLSpdVld','40','2','BE','unsigned','Standard','0','1','0','-Inf','Inf';'WhlRRSpd','58','14','BE','unsigned','Standard','0','1','0','-Inf','Inf';'WhlRRSpdVld','56','2','BE','unsigned','Standard','0','1','0','-Inf','Inf'}  IDPort=off  TimestampPort=off  ErrorPort=off  RemotePort=off  LengthPort=off  StatusPort=off  ApplyMinMax=off
      settings: SourceProductBaseCode=ME,VN  DataFormat=CANdb specified signals
  EHB_WhlFLSpd : DataTypeConversion
  EHB_WhlFLSpdVld : DataTypeConversion
  EHB_WhlFRSpd : DataTypeConversion
  EHB_WhlFRSpdVld : DataTypeConversion
  EHB_WhlRLSpd : DataTypeConversion
  EHB_WhlRLSpdVld : DataTypeConversion
  EHB_WhlRRSpd : DataTypeConversion
  EHB_WhlRRSpdVld : DataTypeConversion
  CAN_Msg_0x127 : Outport
  wires:
  EHB_WhlRLSpdVld/1 -> Bus Creator/6  "EHB_WhlRLSpdVld"
  EHB_WhlRLSpd/1 -> Bus Creator/5  "EHB_WhlRLSpd"
  EHB_WhlFRSpdVld/1 -> Bus Creator/4  "EHB_WhlFRSpdVld"
  Can Unpack/6 -> EHB_WhlRLSpdVld/1
  Can Unpack/5 -> EHB_WhlRLSpd/1
  Can Unpack/4 -> EHB_WhlFRSpdVld/1
  CAN Msg/1 -> Can Unpack/1
  Can Unpack/1 -> EHB_WhlFLSpd/1
  EHB_WhlFLSpd/1 -> Bus Creator/1  "EHB_WhlFLSpd"
  Can Unpack/2 -> EHB_WhlFLSpdVld/1
  EHB_WhlFLSpdVld/1 -> Bus Creator/2  "EHB_WhlFLSpdVld"
  Can Unpack/3 -> EHB_WhlFRSpd/1
  EHB_WhlFRSpd/1 -> Bus Creator/3  "EHB_WhlFRSpd"
  Bus Creator/1 -> CAN_Msg_0x127/1  "CAN_Msg_0x127"
  Can Unpack/7 -> EHB_WhlRRSpd/1
  Can Unpack/8 -> EHB_WhlRRSpdVld/1
  EHB_WhlRRSpd/1 -> Bus Creator/7  "EHB_WhlRRSpd"
  EHB_WhlRRSpdVld/1 -> Bus Creator/8  "EHB_WhlRRSpdVld"

== system EHB_speedgoat_R2020a_V1/CAN_Rec/CAN Receive/Debug1_0x287 ==
  CAN Msg : Inport
  Enable : EnablePort
  Bus Creator : BusCreator  Inputs=4
  Can Unpack : canmsglib/CAN Unpack  CANdbFile=F:\湖大艾盛\wushuadianji_20230612.dbc  MsgList=Debug1  MsgName=Debug1  MsgIDType=Standard (11-bit identifier)  MsgIdentifier=647  MsgLength=8  SignalInfo={'iBeta','8','16','BE','signed','Standard','0','0.01','0','-Inf','Inf';'ia_ADC','40','16','BE','unsigned','Standard','0','1','0','-Inf','Inf';'ib_ADC','56','16','BE','unsigned','Standard','0','1','0','-Inf','Inf';'sin_theta','24','16','BE','signed','Standard','0','0.001','0','-Inf','Inf'}  IDPort=off  TimestampPort=off  ErrorPort=off  RemotePort=off  LengthPort=off  StatusPort=off  ApplyMinMax=off
      settings: SourceProductBaseCode=ME,VN  DataFormat=CANdb specified signals
  iBeta : DataTypeConversion
  ia_ADC : DataTypeConversion
  ib_ADC : DataTypeConversion
  sin_theta : DataTypeConversion
  Debug1 : Outport
  wires:
  CAN Msg/1 -> Can Unpack/1
  Can Unpack/1 -> iBeta/1
  iBeta/1 -> Bus Creator/1  "iBeta"
  Can Unpack/2 -> ia_ADC/1
  ia_ADC/1 -> Bus Creator/2  "ia_ADC"
  Can Unpack/3 -> ib_ADC/1
  ib_ADC/1 -> Bus Creator/3  "ib_ADC"
  Can Unpack/4 -> sin_theta/1
  sin_theta/1 -> Bus Creator/4  "sin_theta"
  Bus Creator/1 -> Debug1/1  "Debug1"

== system EHB_speedgoat_R2020a_V1/CAN_Rec/CAN Receive/Debug_0x286 ==
  CAN Msg : Inport
  Enable : EnablePort
  Bus Creator : BusCreator  Inputs=4
  Can Unpack : canmsglib/CAN Unpack  CANdbFile=F:\湖大艾盛\wushuadianji_20230612.dbc  MsgList=Debug  MsgName=Debug  MsgIDType=Standard (11-bit identifier)  MsgIdentifier=646  MsgLength=8  SignalInfo={'Ualpha','40','16','BE','signed','Standard','0','1','0','-Inf','Inf';'Ubeta','56','16','BE','signed','Standard','0','1','0','-Inf','Inf';'angle','8','16','BE','unsigned','Standard','0','1','0','-Inf','Inf';'cos_theta','24','16','BE','signed','Standard','0','0.001','0','-Inf','Inf'}  IDPort=off  TimestampPort=off  ErrorPort=off  RemotePort=off  LengthPort=off  StatusPort=off  ApplyMinMax=off
      settings: SourceProductBaseCode=ME,VN  DataFormat=CANdb specified signals
  Ualpha : DataTypeConversion
  Ubeta : DataTypeConversion
  angle : DataTypeConversion
  cos_theta : DataTypeConversion
  Debug : Outport
  wires:
  CAN Msg/1 -> Can Unpack/1
  Can Unpack/1 -> Ualpha/1
  Ualpha/1 -> Bus Creator/1  "Ualpha"
  Can Unpack/2 -> Ubeta/1
  Ubeta/1 -> Bus Creator/2  "Ubeta"
  Can Unpack/3 -> angle/1
  angle/1 -> Bus Creator/3  "angle"
  Can Unpack/4 -> cos_theta/1
  cos_theta/1 -> Bus Creator/4  "cos_theta"
  Bus Creator/1 -> Debug/1  "Debug"

== system EHB_speedgoat_R2020a_V1/CAN_Rec/CAN Receive/Message_1_0x281 ==
  CAN Msg : Inport
  Enable : EnablePort
  Angle1 : DataTypeConversion
  Bus Creator : BusCreator  Inputs=4
  Can Unpack : canmsglib/CAN Unpack  CANdbFile=F:\湖大艾盛\wushuadianji_20230612.dbc  MsgList=Message_1  MsgName=Message_1  MsgIDType=Standard (11-bit identifier)  MsgIdentifier=641  MsgLength=8  SignalInfo={'Angle1','56','16','BE','signed','Standard','0','1','0','-Inf','Inf';'U_Current','8','16','BE','signed','Standard','0','1','0','-Inf','Inf';'V_Current','24','16','BE','signed','Standard','0','1','0','-Inf','Inf';'W_Current','40','16','BE','signed','Standard','0','1','0','-Inf','Inf'}  IDPort=off  TimestampPort=off  ErrorPort=off  RemotePort=off  LengthPort=off  StatusPort=off  ApplyMinMax=off
      settings: SourceProductBaseCode=ME,VN  DataFormat=CANdb specified signals
  U_Current : DataTypeConversion
  V_Current : DataTypeConversion
  W_Current : DataTypeConversion
  Message_1 : Outport
  wires:
  CAN Msg/1 -> Can Unpack/1
  Can Unpack/1 -> Angle1/1
  Angle1/1 -> Bus Creator/1  "Angle1"
  Can Unpack/2 -> U_Current/1
  U_Current/1 -> Bus Creator/2  "U_Current"
  Can Unpack/3 -> V_Current/1
  V_Current/1 -> Bus Creator/3  "V_Current"
  Can Unpack/4 -> W_Current/1
  W_Current/1 -> Bus Creator/4  "W_Current"
  Bus Creator/1 -> Message_1/1  "Message_1"

== system EHB_speedgoat_R2020a_V1/CAN_Rec/CAN Receive/Message_2_0x282 ==
  CAN Msg : Inport
  Enable : EnablePort
  Angle2 : DataTypeConversion
  Bus Creator : BusCreator  Inputs=4
  Can Unpack : canmsglib/CAN Unpack  CANdbFile=F:\湖大艾盛\wushuadianji_20230612.dbc  MsgList=Message_2  MsgName=Message_2  MsgIDType=Standard (11-bit identifier)  MsgIdentifier=642  MsgLength=8  SignalInfo={'Angle2','8','16','BE','signed','Standard','0','1','0','-Inf','Inf';'U_DutyCycle','24','16','BE','signed','Standard','0','1','0','-Inf','Inf';'V_DutyCycle','40','16','BE','signed','Standard','0','1','0','-Inf','Inf';'W_DutyCycle','56','16','BE','signed','Standard','0','1','0','-Inf','Inf'}  IDPort=off  TimestampPort=off  ErrorPort=off  RemotePort=off  LengthPort=off  StatusPort=off  ApplyMinMax=off
      settings: SourceProductBaseCode=ME,VN  DataFormat=CANdb specified signals
  U_DutyCycle : DataTypeConversion
  V_DutyCycle : DataTypeConversion
  W_DutyCycle : DataTypeConversion
  Message_2 : Outport
  wires:
  CAN Msg/1 -> Can Unpack/1
  Can Unpack/1 -> Angle2/1
  Angle2/1 -> Bus Creator/1  "Angle2"
  Can Unpack/2 -> U_DutyCycle/1
  U_DutyCycle/1 -> Bus Creator/2  "U_DutyCycle"
  Can Unpack/3 -> V_DutyCycle/1
  V_DutyCycle/1 -> Bus Creator/3  "V_DutyCycle"
  Can Unpack/4 -> W_DutyCycle/1
  W_DutyCycle/1 -> Bus Creator/4  "W_DutyCycle"
  Bus Creator/1 -> Message_2/1  "Message_2"

== system EHB_speedgoat_R2020a_V1/CAN_Rec/CAN Receive/Message_3_0x283 ==
  CAN Msg : Inport
  Enable : EnablePort
  Bus Creator : BusCreator  Inputs=2
  Can Unpack : canmsglib/CAN Unpack  CANdbFile=F:\湖大艾盛\wushuadianji_20230612.dbc  MsgList=Message_3  MsgName=Message_3  MsgIDType=Standard (11-bit identifier)  MsgIdentifier=643  MsgLength=8  SignalInfo={'ia_act','24','32','BE','signed','Standard','0','1','0','-Inf','Inf';'ib_act','56','32','BE','signed','Standard','0','1','0','-Inf','Inf'}  IDPort=off  TimestampPort=off  ErrorPort=off  RemotePort=off  LengthPort=off  StatusPort=off  ApplyMinMax=off
      settings: SourceProductBaseCode=ME,VN  DataFormat=CANdb specified signals
  ia_act : DataTypeConversion
  ib_act : DataTypeConversion
  Message_3 : Outport
  wires:
  CAN Msg/1 -> Can Unpack/1
  Can Unpack/1 -> ia_act/1
  ia_act/1 -> Bus Creator/1  "ia_act"
  Can Unpack/2 -> ib_act/1
  ib_act/1 -> Bus Creator/2  "ib_act"
  Bus Creator/1 -> Message_3/1  "Message_3"

== system EHB_speedgoat_R2020a_V1/CAN_Rec/CAN Receive/Message_4_0x284 ==
  CAN Msg : Inport
  Enable : EnablePort
  Bus Creator : BusCreator  Inputs=4
  Can Unpack : canmsglib/CAN Unpack  CANdbFile=F:\湖大艾盛\wushuadianji_20230612.dbc  MsgList=Message_4  MsgName=Message_4  MsgIDType=Standard (11-bit identifier)  MsgIdentifier=644  MsgLength=8  SignalInfo={'MOTOR_ID','24','16','BE','signed','Standard','0','0.01','0','-Inf','Inf';'MOTOR_IQ','40','16','BE','signed','Standard','0','0.01','0','-Inf','Inf';'PWM_Duty_Group0_2','8','16','BE','unsigned','Standard','0','0.013333','0','-Inf','Inf';'iAlpha','56','16','BE','signed','Standard','0','0.01','0','-Inf','Inf'}  IDPort=off  TimestampPort=off  ErrorPort=off  RemotePort=off  LengthPort=off  StatusPort=off  ApplyMinMax=off
      settings: SourceProductBaseCode=ME,VN  DataFormat=CANdb specified signals
  MOTOR_ID : DataTypeConversion
  MOTOR_IQ : DataTypeConversion
  PWM_Duty_Group0_2 : DataTypeConversion
  iAlpha : DataTypeConversion
  Message_4 : Outport
  wires:
  CAN Msg/1 -> Can Unpack/1
  Can Unpack/1 -> MOTOR_ID/1
  MOTOR_ID/1 -> Bus Creator/1  "MOTOR_ID"
  Can Unpack/2 -> MOTOR_IQ/1
  MOTOR_IQ/1 -> Bus Creator/2  "MOTOR_IQ"
  Can Unpack/3 -> PWM_Duty_Group0_2/1
  PWM_Duty_Group0_2/1 -> Bus Creator/3  "PWM_Duty_Group0_2"
  Can Unpack/4 -> iAlpha/1
  iAlpha/1 -> Bus Creator/4  "iAlpha"
  Bus Creator/1 -> Message_4/1  "Message_4"

== system EHB_speedgoat_R2020a_V1/CAN_Rec/CAN Receive/Message_5_0x285 ==
  CAN Msg : Inport
  Enable : EnablePort
  Bus Creator : BusCreator  Inputs=3
  Can Unpack : canmsglib/CAN Unpack  CANdbFile=F:\湖大艾盛\wushuadianji_20230612.dbc  MsgList=Message_5  MsgName=Message_5  MsgIDType=Standard (11-bit identifier)  MsgIdentifier=645  MsgLength=8  SignalInfo={'PWM_Duty_Group0_0','40','16','BE','unsigned','Standard','0','0.013333','0','-Inf','Inf';'PWM_Duty_Group0_1','56','16','BE','unsigned','Standard','0','0.013333','0','0','873.8';'veelspeed','24','32','BE','signed','Standard','0','0.16667','0','-Inf','Inf'}  IDPort=off  TimestampPort=off  ErrorPort=off  RemotePort=off  LengthPort=off  StatusPort=off  ApplyMinMax=off
      settings: SourceProductBaseCode=ME,VN  DataFormat=CANdb specified signals
  PWM_Duty_Group0_0 : DataTypeConversion
  PWM_Duty_Group0_1 : DataTypeConversion
  veelspeed : DataTypeConversion
  Message_5 : Outport
  wires:
  CAN Msg/1 -> Can Unpack/1
  Can Unpack/1 -> PWM_Duty_Group0_0/1
  PWM_Duty_Group0_0/1 -> Bus Creator/1  "PWM_Duty_Group0_0"
  Can Unpack/2 -> PWM_Duty_Group0_1/1
  PWM_Duty_Group0_1/1 -> Bus Creator/2  "PWM_Duty_Group0_1"
  Can Unpack/3 -> veelspeed/1
  veelspeed/1 -> Bus Creator/3  "veelspeed"
  Bus Creator/1 -> Message_5/1  "Message_5"

== system EHB_speedgoat_R2020a_V1/CAN_Send/CAN Transmit/VCU_Msg ==
  Trigger : Inport
  VCU_Msg : Inport  Port=2
  Enable : EnablePort
  Bus Selector : BusSelector  OutputSignals=Trigger_VCU_BrakingRequest_0x120,Enable_VCU_BrakingRequest_0x120
  Bus Selector1 : BusSelector  OutputSignals=VCU_BrakingRequest_0x120
  VCU_BrakingRequest_0x120 : Subsystem  TreatAsAtomicUnit=on
  wires:
  Trigger/1 -> Bus Selector/1
  Bus Selector/1 -> VCU_BrakingRequest_0x120/Trigger  "<Trigger_VCU_BrakingRequest_0x120>"
  Bus Selector/2 -> VCU_BrakingRequest_0x120/Enable  "<Enable_VCU_BrakingRequest_0x120>"
  Bus Selector1/1 -> VCU_BrakingRequest_0x120/1(VCU_BrakingRequest)  "<VCU_BrakingRequest_0x120>"
  VCU_Msg/1 -> Bus Selector1/1

== system EHB_speedgoat_R2020a_V1/CAN_Send/Signal/CAN_Msg_VCU ==
  Bus Creator : BusCreator  Inputs=1
  VCU_BrakingRequest_0x120 : Subsystem
  VCU_Msg : Outport
  wires:
  VCU_BrakingRequest_0x120/1(VCU_BrakingRequest_0x120) -> Bus Creator/1  "VCU_BrakingRequest_0x120"
  Bus Creator/1 -> VCU_Msg/1  "VCU_Msg"

== system EHB_speedgoat_R2020a_V1/CAN_Send/Trigger/Trigger_VCU_Msg ==
  Bus Creator : BusCreator  Inputs=3
  Enable_VCU_BrakingRequest_0x120 : Constant
  Enable_VCU_Msg : Constant
  Trigger_VCU_BrakingRequest_0x120 : Subsystem  mask(Cansend trigger mode selection){ModeSelect=1, EnablePeriod=0.001, Period=50, MsgLstCnt=0}
      mask prompts: EnablePeriod "EnablePeriod(s)"; Period "Period(ms)"
      mask help:
      | ModeSelect value description :
      | 1:period of transmission
      | 2: manually send
      | 3:conditional trigger
      mask TypeOptions ModeSelect: 1 | 2 | 3
      mask Callback ModeSelect:
      | mode = get(gcbh,'ModeSelect');
      | 
      | if(mode == '3')
      |     if(isempty(find_system(gcb,'LookUnderMasks','on','SearchDepth',1,'BlockType','Inport')))
      |         path = get(gcbh,'Path');
      |         name = get(gcbh,'Name');
      |         find_system(gcbh,'block','');
      |         inportsource  = 'simulink/Sources/In1';
      |         inportdist = [path,'/',name,'/','ConditionalTrigger'];
      |         handle_tmp = find_system(gcbh,'name','ConditionalTrigger');
      |         position_tmp = get_param(inportdist,'Position');
      | 
      |         delete_block(inportdist);
      |         add_block(inportsource,inportdist,'Position',position_tmp);
      | 
      |     else
      | 
      |     end
      | else
      |     path = get(gcbh,'Path');
      |     name = get(gcbh,'Name');
      |     find_system(gcbh,'block','');
      |     inportsource  = 'simulink/Sources/Ground';
      |     inportdist = [path,'/',name,'/','ConditionalTrigger'];
      |     handle_tmp = find_system(gcbh,'name','ConditionalTrigger');
      |     position_tmp = get_param(inportdist,'Position');
      | 
      |     delete_block(inportdist);
      |     add_block(inportsource,inportdist,'Position',position_tmp);
      | 
      | 
      | end
      mask Display:
      | plot([0 0.3 0.3 0.7 0.7 1],[0.1 0.1 0.8 0.8 0.1 0.1]);
      | port_label('output', 1, 'CndTriggerout');
      | if(isempty(find_system(gcb,'LookUnderMasks','on','SearchDepth',1,'BlockType','Inport')))
      | else
      |    port_label('input', 1, 'CndTriggerin');
      | end
  VCU_Msg : Outport
  wires:
  Enable_VCU_BrakingRequest_0x120/1 -> Bus Creator/1  "Enable_VCU_BrakingRequest_0x120"
  Trigger_VCU_BrakingRequest_0x120/1(Out1) -> Bus Creator/2  "Trigger_VCU_BrakingRequest_0x120"
  Enable_VCU_Msg/1 -> Bus Creator/3  "Enable_VCU_Msg"
  Bus Creator/1 -> VCU_Msg/1  "VCU_Msg"

== system EHB_speedgoat_R2020a_V1/PowerCtrl/PowerCtrl/CANOpenInit1 ==
  Start/Stop : Inport
  CAN Pack : canmsglib/CAN Pack  MsgList=(none)  MsgName=CAN Msg  MsgIDType=Standard (11-bit identifier)  MsgIdentifier=0  MsgLength=2  Remote=off  ApplyMinMax=off  BusOutput=on  SignalInfo={}
      settings: SourceProductBaseCode=ME,VN  DataFormat=raw data
  CANDataPack_ToUDP : Subsystem
  ID : Constant  OutDataTypeStr=uint8
  Mux : Mux  Inputs=2
  Start : Constant  OutDataTypeStr=Inherit: Inherit via back propagation
  Stop : Constant  Value=2  OutDataTypeStr=Inherit: Inherit via back propagation
  Switch : Switch  Criteria=u2 > Threshold  OutDataTypeStr=uint8
  Output : Outport
  wires:
  Stop/1 -> Switch/3
  Start/1 -> Switch/1
  Switch/1 -> Mux/1
  Start/Stop/1 -> Switch/2
  CAN Pack/1 -> CANDataPack_ToUDP/1(In1)
  Mux/1 -> CAN Pack/1
  ID/1 -> Mux/2
  CANDataPack_ToUDP/1(Output) -> Output/1
